simulink model "s0524"  (Simulink 7.0)
settings: Solver=ode45  SolverMode=SingleTasking  StartTime=0.0  StopTime=999999  MaxStep=10  RelTol=1e-3  AbsTol=1e-6
values from neighbouring files (symbols this model uses):
  Kpr = 10    [m0108d.m]    (also in m0109b.m = 1; m0113c.m; m0404Bsp.m = 3)
  wdach = 0    [m0109b.m]    (also in m0404Bsp.m = 1)
undefined symbols (not defined in the file or in its folder): Kv, rnen, rzae, snen, szae, tstep
settings Model: Creator=froriep  LastModifiedBy=froriep
settings DataIOCC: LimitDataPoints=off  SaveOutput=off  SaveTime=off
settings OptimizationCC: BooleanDataType=off  InlineInvariantSignals=on
settings DebuggingCC: SaveWithParameterizedLinksMsg=none  SignalResolutionControl=TryResolveAllWithWarning  SolverPrmCheckMsg=none  MultiTaskDSMMsg=warning  MultiTaskCondExecSysMsg=none  StrictBusMsg=None
settings HardwareCC: TargetUnknown=on
settings RTWCC: IncludeERTFirstTime=on
settings GRTTargetCC: TargetFcnLib=ansi_tfl_tmw.mat  ModelReferenceCompliant=off  CompOptLevelCompliant=off  MatFileLogging=off

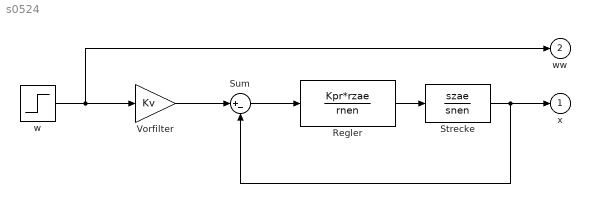
== system s0524 ==
  Regler : TransferFcn  Numerator=Kpr*rzae  Denominator=rnen
  Strecke : TransferFcn  Numerator=szae  Denominator=snen
  Sum : Sum  Inputs=|+-  OutDataType=sfix(16)  OutScaling=2^0  SaturateOnIntegerOverflow=on  InputSameDT=on
  Vorfilter : Gain  Gain=Kv  ParameterDataType=sfix(16)  ParameterScaling=2^0  OutDataType=sfix(16)  OutScaling=2^0  SaturateOnIntegerOverflow=on
  w : Step  Time=tstep  After=wdach  SampleTime=0
  x : Outport  OutDataType=sfix(16)  OutScaling=2^0
  ww : Outport  Port=2  OutDataType=sfix(16)  OutScaling=2^0
  wires:
  w/1 -> ww/1, Vorfilter/1
  Vorfilter/1 -> Sum/1
  Strecke/1 -> Sum/2, x/1
  Sum/1 -> Regler/1
  Regler/1 -> Strecke/1
